simulink model "controller_testing_model_prev"  (R2015a)
settings: Solver=ode45  StartTime=0.0  StopTime=10.0  RelTol=1e-3
undefined symbols (not defined in the file): A, B, C, D, K, M, Nbar, x_init
settings Model: Creator=Alunos  LastModifiedBy=Alunos

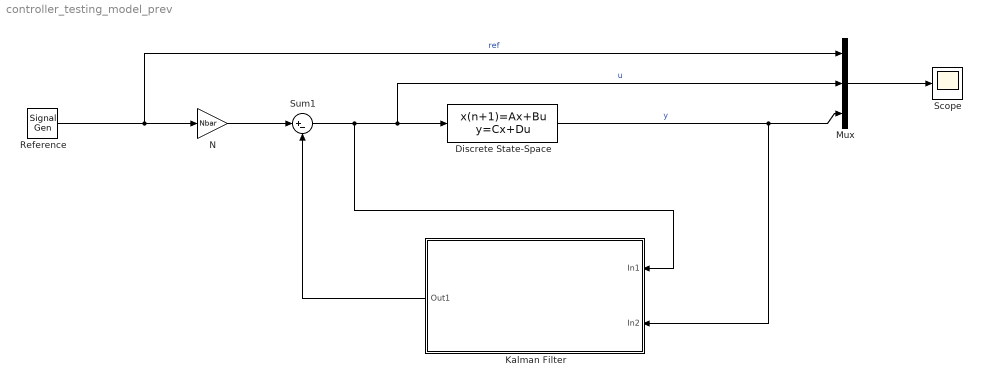
== system controller_testing_model_prev ==
  Discrete State-Space : DiscreteStateSpace  A=A  B=B  C=C  D=D  X0=x_init  SampleTime=0.002
  Kalman Filter : Subsystem
  Mux : Mux  Inputs=3
  N : Gain  Gain=Nbar
  Reference : SignalGenerator  WaveForm=square  Amplitude=0.5  Frequency=0.4
  Scope : Scope
      settings: ShowLegends=on
  Sum1 : Sum  Inputs=|+-
  wires:
  Sum1/1 -> Kalman Filter/1(In1), Mux/2, Discrete State-Space/1  "u"
  N/1 -> Sum1/1
  Discrete State-Space/1 -> Kalman Filter/2(In2), Mux/3  "y"
  Kalman Filter/1(Out1) -> Sum1/2
  Reference/1 -> Mux/1, N/1  "ref"
  Mux/1 -> Scope/1

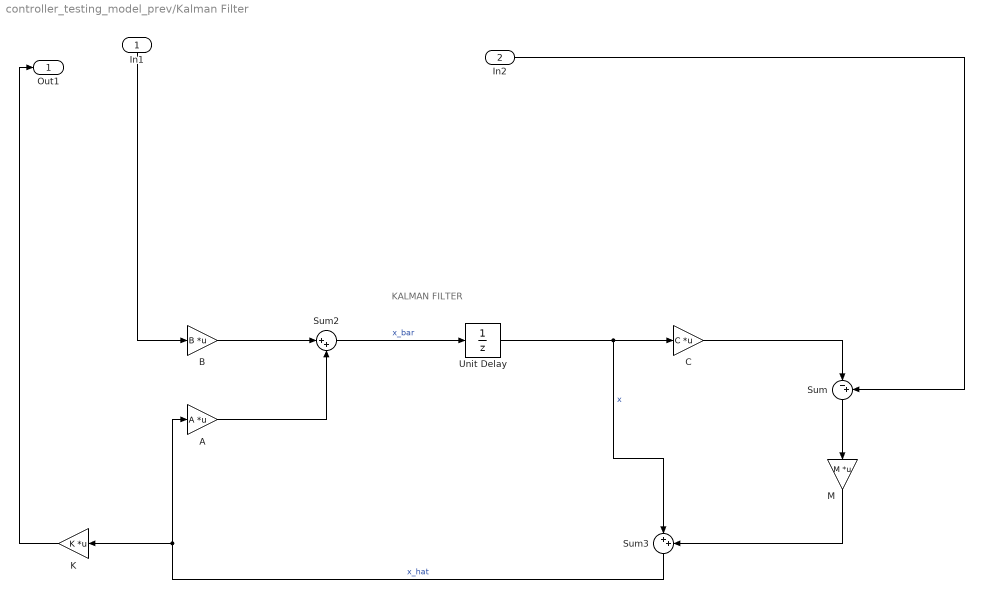
== system controller_testing_model_prev/Kalman Filter ==
  note: KALMAN FILTER
  In1 : Inport
  In2 : Inport  Port=2
  A : Gain  Gain=A  Multiplication=Matrix(K*u)
  B : Gain  Gain=B  Multiplication=Matrix(K*u)
  C : Gain  Gain=C  Multiplication=Matrix(K*u)
  K : Gain  Gain=K  Multiplication=Matrix(K*u)
  M : Gain  Gain=M  Multiplication=Matrix(K*u)
  Sum : Sum  Inputs=|-+
  Sum2 : Sum  Inputs=|++
  Sum3 : Sum  Inputs=|++
  Unit Delay : UnitDelay  InitialCondition=x_init  SampleTime=-1
  Out1 : Outport
  wires:
  M/1 -> Sum3/2
  Sum2/1 -> Unit Delay/1  "x_bar"
  A/1 -> Sum2/2
  B/1 -> Sum2/1
  Sum3/1 -> A/1, K/1  "x_hat"
  Sum/1 -> M/1
  In2/1 -> Sum/2
  C/1 -> Sum/1
  Unit Delay/1 -> C/1, Sum3/1  "x"
  K/1 -> Out1/1
  In1/1 -> B/1
